simulink model "IndustrialMicrogrid"  (R2023a)
settings: Solver=FixedStepDiscrete  StartTime=0.0  StopTime=10  FixedStep=Ts  RelTol=1e-3
PostLoadFcn:
  | IndustrialMicrogridInputData
  | GfmGridFormingConverterInputParameters
model workspace (MAT data in the model file):
  caseNum = 2
undefined symbols (not defined in the file): base, BESS, DiscIntNeverNeededParam, grid, Grid, gridInverter, machine, microgrid, PV, PVInverter, PVTransformer, scrFactorRg, scrFactorXg, transformer, Ts
libraries: ee_lib x112, eeGeneralControl x104, nesl_utility_internal x64, simulink x56, nesl_utility x37, fl_lib x29, slpidlib x13, eeTransforms x11, eeTotalHarmonicDistorsion x8, eeRmsMeasurement x4, eeSinusoidalMeasurement x4, simulink_extras x2
(part 12 of 14)

== system IndustrialMicrogrid/MG2 Primary Substation/BESS and Controller 2/BESS/Grid-Forming Converter Control/Grid Voltage Reactive Power Support/Modifying Reactive Power Reference/Changing the Power Reference ==
  Vs : Inport
  Vd : Inport  Port=2
  Pref : Inport  Port=3
  Qref : Inport  Port=4
  Enable : EnablePort
  ActivePowerReference : Subsystem
  Constant1 : Constant  Value=voltreference*0.96
  EstimateIdForGivenIq : Subsystem
  EstimateIqForReactivePower : Subsystem
  Max : MinMax  Function=max  Inputs=2
  ReactivePowerReference : Subsystem
  Prefv : Outport
  Qrefv : Outport  Port=2
  wires:
  EstimateIqForReactivePower/1(Iq) -> EstimateIdForGivenIq/1(Iq), ReactivePowerReference/2(Iq)
  Constant1/1 -> EstimateIqForReactivePower/1(Vmin)
  Vs/1 -> ActivePowerReference/2(Vd), EstimateIqForReactivePower/3(Vs), ReactivePowerReference/1(Vd)
  EstimateIdForGivenIq/1(Id) -> ActivePowerReference/1(Id)
  Pref/1 -> ActivePowerReference/3(Pref)
  ActivePowerReference/1(PrefNew) -> Prefv/1
  ReactivePowerReference/1(QrefNew) -> Max/1
  Max/1 -> Qrefv/1
  Qref/1 -> Max/2
  Vd/1 -> EstimateIqForReactivePower/2(Vd)

== system IndustrialMicrogrid/MG2 Primary Substation/BESS and Controller 2/BESS/Grid-Forming Converter Control/Grid Voltage Reactive Power Support/Modifying Reactive Power Reference/Hysteresis ==
  Vs : Inport
  AND : Logic  IconShape=distinctive  AllPortsSameDT=off  OutDataTypeStr=boolean
  Compare To Constant : simulink/Logic and Bit Operations/Compare To Constant  relop=<  const=0.9  OutDataTypeStr=boolean
  Compare To Constant1 : simulink/Logic and Bit Operations/Compare To Constant  relop=<  const=0.95  OutDataTypeStr=boolean
  D Latch : simulink_extras/Flip Flops/D Latch
  OR : Logic  Operator=OR  IconShape=distinctive  AllPortsSameDT=off  OutDataTypeStr=boolean
  Terminator : Terminator
  LVFlag : Outport
  wires:
  Compare To Constant1/1 -> AND/1
  D Latch/1 -> AND/2
  AND/1 -> OR/1
  OR/1 -> LVFlag/1
  D Latch/2 -> Terminator/1
  Compare To Constant/1 -> D Latch/1, D Latch/2, OR/2
  Vs/1 -> Compare To Constant1/1, Compare To Constant/1

== system IndustrialMicrogrid/MG2 Primary Substation/BESS and Controller 2/BESS/Grid-Forming Converter Control/Grid Voltage Reactive Power Support/Modifying Reactive Power Reference/Not Altering the Power Reference ==
  Pref : Inport
  Qref : Inport  Port=2
  Enable : EnablePort
  Prefv : Outport
  Qrefv : Outport  Port=2
  wires:
  Pref/1 -> Prefv/1
  Qref/1 -> Qrefv/1

== system IndustrialMicrogrid/MG2 Primary Substation/BESS and Controller 2/BESS/Grid-Forming Converter Control/Measurement/Frequency Measurement/Frequency Measurement ==
  abc : Inport
  Constant : Constant
  Discrete-Time Integrator : DiscreteIntegrator  SampleTime=sampleTime  LimitOutput=on  ICPrevOutput=DiscIntNeverNeededParam  ICPrevScaledInput=DiscIntNeverNeededParam
  If : If  IfExpression=u1 > 0.9
  If Action Subsystem : Subsystem  TreatAsAtomicUnit=on
  If Action Subsystem1 : Subsystem  TreatAsAtomicUnit=on
  Merge : Merge
  Postive Sequence : Subsystem
  Freq : Outport
  wires:
  If/1 -> If Action Subsystem/Action
  If/2 -> If Action Subsystem1/Action
  Discrete-Time Integrator/1 -> If Action Subsystem/2(Time), If/1
  abc/1 -> Postive Sequence/1(abc)
  Constant/1 -> Discrete-Time Integrator/1
  If Action Subsystem/1(Freq) -> Merge/1
  If Action Subsystem1/1(Out1) -> Merge/2
  Merge/1 -> Freq/1
  Postive Sequence/1(posSeq) -> If Action Subsystem/1(V)

== system IndustrialMicrogrid/MG2 Primary Substation/BESS and Controller 2/BESS/Grid-Forming Converter Control/Measurement/abc2dq/Supply Current to dq ==
  abc : Inport
  Angle : Inport  Port=2
  Demux : Demux  Outputs=3
  Park Transform : eeTransforms/Park Transform  AxisAlignment=D-axis  PowerInvariant=off
  Terminator : Terminator
  Igd : Outport  VectorParamsAs1DForOutWhenUnconnected=off
  Igq : Outport  Port=2  VectorParamsAs1DForOutWhenUnconnected=off
  wires:
  Demux/3 -> Terminator/1
  Park Transform/1 -> Demux/1
  Demux/2 -> Igq/1
  Demux/1 -> Igd/1
  abc/1 -> Park Transform/1
  Angle/1 -> Park Transform/2

== system IndustrialMicrogrid/MG2 Primary Substation/BESS and Controller 2/BESS/Grid-Forming Converter Control/Measurement/abc2dq/Supply Voltage  to dq1 ==
  Angle : Inport
  abc : Inport  Port=2
  Demux : Demux  Outputs=3
  Park Transform : eeTransforms/Park Transform  AxisAlignment=D-axis  PowerInvariant=off
  Terminator : Terminator
  Vgd : Outport  VectorParamsAs1DForOutWhenUnconnected=off
  Vgq : Outport  Port=2  VectorParamsAs1DForOutWhenUnconnected=off
  wires:
  Demux/3 -> Terminator/1
  Park Transform/1 -> Demux/1
  Demux/2 -> Vgq/1
  Demux/1 -> Vgd/1
  abc/1 -> Park Transform/1
  Angle/1 -> Park Transform/2

== system IndustrialMicrogrid/MG2 Primary Substation/BESS and Controller 2/BESS/Grid-Forming Converter Control/Power Control/ActivePowerControl/droopControl ==
  Pref : Inport
  Pmeas : Inport  Port=2
  fref : Inport  Port=3
  cntrlflag : Inport  Port=4
  fgrid : Inport  Port=5
  Add : Sum  Inputs=+-
  Constant : Constant
  Constant5 : Constant  Value=pi/2
  Gain : Gain  Gain=powerFreq*2*pi
  Integrator with Wrapped State (Discrete or Continuous) : eeGeneralControl/Integrator with Wrapped State (Discrete or Continuous)  LabelModeActiveChoice=Discrete  WrappedStateUpperValue=2*pi  WrappedStateLowerValue=0  x0=0  Ts=activePowerSampleTime
      settings: LibrarySourceBlock=|
      | ee_sl_lib/General Control/Integrator with
      | Wrapped State
      | (Discrete or Continuous)
  Lead-Lag (Discrete or Continuous) : eeGeneralControl/Lead-Lag (Discrete or Continuous)  T1=droopT1  T2=droopT2  B=inf  A=-inf  init_option=Inherited from block input  x0=0  Ts=activePowerSampleTime
      settings: LibrarySourceBlock=|
      | ee_sl_lib/General Control/Lead-Lag
      | (Discrete or Continuous)
  Low-Pass Filter (Discrete or Continuous) : eeGeneralControl/Low-Pass Filter (Discrete or Continuous)  K=1  T=droopTC  B=inf  A=-inf  init_option=Specify as parameter  x0=0  Ts=activePowerSampleTime
  Sum : Sum  Inputs=|-+
  Sum1 : Sum  Inputs=|-+
  Terminator : Terminator
  Terminator1 : Terminator
  Terminator2 : Terminator
  mp : Gain  Gain=droopSlope
  Theta : Outport
  w : Outport  Port=2
  wires:
  Low-Pass Filter (Discrete or Continuous)/1 -> Sum1/1
  mp/1 -> Low-Pass Filter (Discrete or Continuous)/1
  Sum/1 -> mp/1
  Pmeas/1 -> Lead-Lag (Discrete or Continuous)/1
  Add/1 -> Theta/1
  Constant5/1 -> Add/2
  Pref/1 -> Sum/1
  Gain/1 -> Integrator with Wrapped State (Discrete or Continuous)/1, w/1
  Lead-Lag (Discrete or Continuous)/1 -> Sum/2
  Integrator with Wrapped State (Discrete or Continuous)/1 -> Add/1
  Constant/1 -> Sum1/2
  Sum1/1 -> Gain/1
  fgrid/1 -> Terminator/1
  fref/1 -> Terminator1/1
  cntrlflag/1 -> Terminator2/1

== system IndustrialMicrogrid/MG2 Primary Substation/BESS and Controller 2/BESS/Grid-Forming Converter Control/Power Control/ActivePowerControl/vsmControl ==
  note: Measured power
  note: Damping power input
  Pref : Inport
  Pmeas : Inport  Port=2
  fref : Inport  Port=3
  cntrlflag : Inport  Port=4
  fgrid : Inport  Port=5
  Add : Sum  Inputs=+-
  Constant2 : Constant  Value=pi/2
  Damping Frequency : Subsystem  Variant=on  VariantControlMode=label  VariantControl=Choice  LabelModeActiveChoice=constFreq
  Discrete-Time Integrator : DiscreteIntegrator  IntegratorMethod=Integration: Backward Euler  InitialCondition=1  SampleTime=activePowerSampleTime  LimitOutput=on  UpperSaturationLimit=1.1  LowerSaturationLimit=0.9  ICPrevOutput=DiscIntNeverNeededParam  ICPrevScaledInput=DiscIntNeverNeededParam
  Gain : Gain  Gain=powerFreq*2*pi
  Gain1 : Gain  Gain=1/vsmInertiaTC
  Gain2 : Gain  Gain=vsmDampingConst*powerFreq
  Integrator with Wrapped State (Discrete or Continuous) : eeGeneralControl/Integrator with Wrapped State (Discrete or Continuous)  LabelModeActiveChoice=Discrete  WrappedStateUpperValue=2*pi  WrappedStateLowerValue=0  x0=0  Ts=activePowerSampleTime
      settings: LibrarySourceBlock=|
      | ee_sl_lib/General Control/Integrator with
      | Wrapped State
      | (Discrete or Continuous)
  Low-Pass Filter (Discrete or Continuous) : eeGeneralControl/Low-Pass Filter (Discrete or Continuous)  K=1  T=vsmPmeasFilterTC  B=inf  A=-inf  init_option=Specify as parameter  x0=0  Ts=activePowerSampleTime
  Power Reference Selection : Subsystem
  Saturation : Saturate  UpperLimit=dampingPowerMaxLimit  LowerLimit=dampingPowerMinLimit
  Sum1 : Sum  Inputs=-+-|
  Sum2 : Sum  Inputs=|+-
  Unit Delay : UnitDelay  SampleTime=-1  HasFrameUpgradeWarning=on
  Unit Delay1 : UnitDelay  SampleTime=-1  HasFrameUpgradeWarning=on
  Theta : Outport
  w : Outport  Port=2
  wires:
  Integrator with Wrapped State (Discrete or Continuous)/1 -> Add/1
  Sum1/1 -> Gain1/1  "Pinertia"
  Constant2/1 -> Add/2
  Add/1 -> Theta/1
  Discrete-Time Integrator/1 -> Gain/1, Unit Delay1/1, Sum2/1
  Low-Pass Filter (Discrete or Continuous)/1 -> Sum1/1
  Gain2/1 -> Saturation/1
  Power Reference Selection/1(power) -> Sum1/2
  Sum2/1 -> Unit Delay/1
  Gain1/1 -> Discrete-Time Integrator/1
  Gain/1 -> Integrator with Wrapped State (Discrete or Continuous)/1, w/1
  Unit Delay/1 -> Gain2/1
  Unit Delay1/1 -> [Wsm]
  Saturation/1 -> Sum1/3  "Pdamping"
  fgrid/1 -> Damping Frequency/1(fref)
  Damping Frequency/1(fmeas) -> Sum2/2
  cntrlflag/1 -> Power Reference Selection/1(cntrlflag)
  Pref/1 -> Power Reference Selection/2(Pref)
  fref/1 -> Power Reference Selection/3(fref)
  Pmeas/1 -> Low-Pass Filter (Discrete or Continuous)/1
  [Wsm] -> Power Reference Selection/4(Wsm)

== system IndustrialMicrogrid/MG2 Primary Substation/BESS and Controller 2/BESS/Grid-Forming Converter Control/Power Control/ReactiveControl/Voltage  Reference Selection ==
  cntrlflag : Inport
  Qref : Inport  Port=2
  Qmeas : Inport  Port=3
  Vref : Inport  Port=4
  Vgdmeas : Inport  Port=5
  If : If
  If Action Subsystem : Subsystem  TreatAsAtomicUnit=on
  If Action Subsystem1 : Subsystem  TreatAsAtomicUnit=on
  Merge : Merge
  Rate Transition : RateTransition
  Vd : Outport
  wires:
  If/1 -> If Action Subsystem/Action
  If Action Subsystem/1(Vd) -> Merge/1
  If/2 -> If Action Subsystem1/Action
  cntrlflag/1 -> Rate Transition/1
  Merge/1 -> Vd/1
  Qmeas/1 -> If Action Subsystem/2(Qmeas)
  Qref/1 -> If Action Subsystem/1(Qref)
  If Action Subsystem1/1(Voltage) -> Merge/2
  Vref/1 -> If Action Subsystem1/1(Vref)
  Vgdmeas/1 -> If Action Subsystem1/2(Vmeas)
  Rate Transition/1 -> If/1

== system IndustrialMicrogrid/MG2 Primary Substation/BESS and Controller 2/BESS/Grid-Forming Converter Control/VoltageCurrentControl/Controller/Id Current Limiting ==
  Imax : Inport
  Id : Inport  Port=2
  Abs : Abs  SaturateOnIntegerOverflow=off
  Switch : Switch  Criteria=u2 > Threshold  SaturateOnIntegerOverflow=off  InputSameDT=off
  Idref : Outport
  wires:
  Id/1 -> Switch/3
  Abs/1 -> Switch/2
  Imax/1 -> Abs/1, Switch/1
  Switch/1 -> Idref/1

== system IndustrialMicrogrid/MG2 Primary Substation/BESS and Controller 2/BESS/Grid-Forming Converter Control/VoltageCurrentControl/Controller/Iq Current Limiting ==
  Imax : Inport
  Iq : Inport  Port=2
  Abs : Abs  SaturateOnIntegerOverflow=off
  Switch : Switch  Criteria=u2 > Threshold  SaturateOnIntegerOverflow=off  InputSameDT=off
  Iqref : Outport
  wires:
  Iq/1 -> Switch/3
  Abs/1 -> Switch/2
  Imax/1 -> Abs/1, Switch/1
  Switch/1 -> Iqref/1

== system IndustrialMicrogrid/MG2 Primary Substation/BESS and Controller 2/BESS/Grid-Forming Converter Control/VoltageCurrentControl/Controller/Voltage control ==
  e : Inport
  resetBlackStart : Inport  Port=2
  Discrete-Time Integrator : DiscreteIntegrator  IntegratorMethod=Integration: Backward Euler  ExternalReset=level  SampleTime=voltControlTs  LimitOutput=on  UpperSaturationLimit=VdMaxCt  LowerSaturationLimit=VdMinCt  ICPrevOutput=DiscIntNeverNeededParam  ICPrevScaledInput=DiscIntNeverNeededParam
  Ki : Gain  Gain=VdIGain
  Kp : Gain  Gain=vdPGain
  Limit : Saturate  UpperLimit=VdMaxCt  LowerLimit=VdMinCt
  Sum7 : Sum  Inputs=|++
  u : Outport  VectorParamsAs1DForOutWhenUnconnected=off
  wires:
  Discrete-Time Integrator/1 -> Sum7/2
  Kp/1 -> Sum7/1
  Limit/1 -> u/1
  Ki/1 -> Discrete-Time Integrator/1
  Sum7/1 -> Limit/1
  e/1 -> Kp/1, Ki/1
  resetBlackStart/1 -> Discrete-Time Integrator/2

== system IndustrialMicrogrid/MG2 Primary Substation/BESS and Controller 2/BESS/Grid-Forming Converter Control/VoltageCurrentControl/Controller/Voltage control1 ==
  e : Inport
  resetBlackStart : Inport  Port=2
  Discrete-Time Integrator : DiscreteIntegrator  IntegratorMethod=Integration: Backward Euler  ExternalReset=level  SampleTime=voltControlTs  LimitOutput=on  UpperSaturationLimit=VqMaxCt  LowerSaturationLimit=VqMinCt  ICPrevOutput=DiscIntNeverNeededParam  ICPrevScaledInput=DiscIntNeverNeededParam
  Ki : Gain  Gain=VqIGain
  Kp : Gain  Gain=VqPGain
  Limit : Saturate  UpperLimit=VqMaxCt  LowerLimit=VqMinCt
  Sum7 : Sum  Inputs=|++
  u : Outport  VectorParamsAs1DForOutWhenUnconnected=off
  wires:
  Discrete-Time Integrator/1 -> Sum7/2
  Sum7/1 -> Limit/1
  e/1 -> Ki/1, Kp/1
  Kp/1 -> Sum7/1
  Ki/1 -> Discrete-Time Integrator/1
  Limit/1 -> u/1
  resetBlackStart/1 -> Discrete-Time Integrator/2

== system IndustrialMicrogrid/MG2 Primary Substation/BESS and Controller 2/BESS/Grid-Forming Converter Control/VoltageCurrentControl/Controller/d-axis current control ==
  e : Inport
  resetBlackStart : Inport  Port=2
  Discrete-Time Integrator : DiscreteIntegrator  IntegratorMethod=Integration: Backward Euler  ExternalReset=level  SampleTime=currentControlTs  LimitOutput=on  UpperSaturationLimit=4  LowerSaturationLimit=-4  ICPrevOutput=DiscIntNeverNeededParam  ICPrevScaledInput=DiscIntNeverNeededParam
  Ki : Gain  Gain=IdIGain
  Kp : Gain  Gain=IdPGain
  Limit : Saturate  UpperLimit=4  LowerLimit=-4
  Sum7 : Sum  Inputs=|++
  u : Outport  VectorParamsAs1DForOutWhenUnconnected=off
  wires:
  Discrete-Time Integrator/1 -> Sum7/2
  Sum7/1 -> Limit/1
  e/1 -> Ki/1, Kp/1
  Kp/1 -> Sum7/1
  Limit/1 -> u/1
  Ki/1 -> Discrete-Time Integrator/1
  resetBlackStart/1 -> Discrete-Time Integrator/2

== system IndustrialMicrogrid/MG2 Primary Substation/BESS and Controller 2/BESS/Grid-Forming Converter Control/VoltageCurrentControl/Controller/q-axis current control ==
  e : Inport
  resetBlackStart : Inport  Port=2
  Discrete-Time Integrator : DiscreteIntegrator  IntegratorMethod=Integration: Backward Euler  ExternalReset=level  SampleTime=currentControlTs  LimitOutput=on  UpperSaturationLimit=3  LowerSaturationLimit=-3  ICPrevOutput=DiscIntNeverNeededParam  ICPrevScaledInput=DiscIntNeverNeededParam
  Ki : Gain  Gain=IqIGain
  Kp : Gain  Gain=IqPGain
  Limit : Saturate  UpperLimit=3  LowerLimit=-3
  Sum7 : Sum  Inputs=|++
  u : Outport  VectorParamsAs1DForOutWhenUnconnected=off
  wires:
  Ki/1 -> Discrete-Time Integrator/1
  Kp/1 -> Sum7/1
  e/1 -> Kp/1, Ki/1
  Sum7/1 -> Limit/1
  Limit/1 -> u/1
  Discrete-Time Integrator/1 -> Sum7/2
  resetBlackStart/1 -> Discrete-Time Integrator/2

== system IndustrialMicrogrid/Operator Room/OperatorControlRoom/MG1 Controller : Commands and Measurements/Microgrid Controller 1 : Commands and Measurements/Measurements and visualizations /BESS, PV and Load Measurements/Active and reactive Power ==
  Grid Active Power : Inport
  BESS Active Power : Inport  Port=2
  Load Active Power : Inport  Port=3
  Grid Reactive Power : Inport  Port=4
  BESS Reactive Power : Inport  Port=5
  Load Reactive Power : Inport  Port=6
  Bus Creator : BusCreator  Inputs=3
  Bus Creator1 : BusCreator  Inputs=3
  Power  Measurements : Scope  NumInputPorts=2
  Active Power : Outport
  Reactive Power : Outport  Port=2
  wires:
  BESS Active Power/1 -> Bus Creator/2
  BESS Reactive Power/1 -> Bus Creator1/2
  Bus Creator1/1 -> Reactive Power/1, Power  Measurements/2
  Bus Creator/1 -> Active Power/1, Power  Measurements/1
  Grid Active Power/1 -> Bus Creator/1
  Load Active Power/1 -> Bus Creator/3
  Grid Reactive Power/1 -> Bus Creator1/1
  Load Reactive Power/1 -> Bus Creator1/3

== system IndustrialMicrogrid/Operator Room/OperatorControlRoom/MG1 Controller : Commands and Measurements/Microgrid Controller 1 : Commands and Measurements/Measurements and visualizations /BESS, PV and Load Measurements/BESS and PV Measurements ==
  Vabc : Inport
  Iabc : Inport  Port=2
  BESS Measurements : Scope  NumInputPorts=4
  Iabc1 : InportShadow  Port=2
  "Inverter Active & Reactive Power " : Subsystem
  Vabc1 : InportShadow
  wires:
  "Inverter Active & Reactive Power "/2(Q) -> BESS Measurements/2  "BESS  Reactive Power (pu)"
  Vabc1/1 -> BESS Measurements/3  "BESS Voltage (pu)"
  "Inverter Active & Reactive Power "/1(P) -> BESS Measurements/1  "BESS  Active Power (pu)"
  Iabc/1 -> "Inverter Active & Reactive Power "/2(Iabc)  "BESS Current (pu)"
  Vabc/1 -> "Inverter Active & Reactive Power "/1(Vabc)  "BESS Voltage (pu)"
  Iabc1/1 -> BESS Measurements/4  "BESS Current (pu)"

== system IndustrialMicrogrid/Operator Room/OperatorControlRoom/MG1 Controller : Commands and Measurements/Microgrid Controller 1 : Commands and Measurements/Measurements and visualizations /BESS, PV and Load Measurements/Load Measurements ==
  Load Active Power : Inport
  Load Reactive Power : Inport  Port=2
  Load Current(p.u.) : Inport  Port=3
  Load Voltage (p.u.) : Inport  Port=4
  Load Voltage RMS (p.u.) : Inport  Port=5
  Bus Creator4 : BusCreator  Inputs=2
  Load Measurements : Scope  NumInputPorts=4
  wires:
  Load Current(p.u.)/1 -> Load Measurements/2  "Load Current(p.u.)"
  Bus Creator4/1 -> Load Measurements/1  "Load Active Power (kW) and reactive power (KVAr)"
  Load Reactive Power/1 -> Bus Creator4/2  "Load Reactive Power (KVAr)"
  Load Voltage RMS (p.u.)/1 -> Load Measurements/4  "Load Voltage RMS (p.u.)"
  Load Active Power/1 -> Bus Creator4/1  "Load Active Power (KW)"
  Load Voltage (p.u.)/1 -> Load Measurements/3  "Load Voltage (p.u.)"

== system IndustrialMicrogrid/Operator Room/OperatorControlRoom/MG1 Controller : Commands and Measurements/Microgrid Controller 1 : Commands and Measurements/Measurements and visualizations /Resynchronization and Planned Islanding/Planned Islanding ==
  Grid Frequency : Inport
  Island Frequency : Inport  Port=2
  Grid Current : Inport  Port=3
  Island Voltage : Inport  Port=4
  Grid Voltage1 : Inport  Port=5
  PlannedIslandCommand : Inport  Port=6
  PlannedIsland : Inport  Port=7
  Power Tracking Command : Inport  Port=8
  " Grid and Island Voltage Frequency " : Scope  NumInputPorts=2
  Bus Creator1 : BusCreator  Inputs=2
  Bus Creator2 : BusCreator  Inputs=2
  Bus Creator3 : BusCreator  Inputs=3
  Bus Creator4 : BusCreator  Inputs=2
  "Grid Active & Reactive Power " : Subsystem
  Grid Voltage2 : InportShadow  Port=5
  Planned Islanding PCC voltage,Current : Scope  NumInputPorts=4
  wires:
  Bus Creator4/1 -> Planned Islanding PCC voltage,Current/4
  Bus Creator3/1 -> Planned Islanding PCC voltage,Current/1
  PlannedIslandCommand/1 -> Bus Creator3/1
  Grid Voltage2/1 -> Planned Islanding PCC voltage,Current/3, "Grid Active & Reactive Power "/1(Vabc)  "Grid Voltage"
  "Grid Active & Reactive Power "/2(Q) -> Bus Creator4/2  "Reactive Power (pu)"
  Grid Current/1 -> Planned Islanding PCC voltage,Current/2, "Grid Active & Reactive Power "/2(Iabc)
  "Grid Active & Reactive Power "/1(P) -> Bus Creator4/1  "Active Power (pu)"
  PlannedIsland/1 -> Bus Creator3/2
  Grid Frequency/1 -> Bus Creator1/1  "Grid Frequency"
  Island Frequency/1 -> Bus Creator1/2  "Island Frequency"
  Bus Creator1/1 -> " Grid and Island Voltage Frequency "/1
  Bus Creator2/1 -> " Grid and Island Voltage Frequency "/2
  Grid Voltage1/1 -> Bus Creator2/1  "Grid Voltage"
  Island Voltage/1 -> Bus Creator2/2  "Island Voltage"
  Power Tracking Command/1 -> Bus Creator3/3

== system IndustrialMicrogrid/Operator Room/OperatorControlRoom/MG1 Controller : Commands and Measurements/Microgrid Controller 1 : Commands and Measurements/Measurements and visualizations /Resynchronization and Planned Islanding/Resync ==
  Grid Frequency : Inport
  Island Frequency : Inport  Port=2
  ResynchCommand : Inport  Port=3
  Grid Angle : Inport  Port=4
  Island Angle : Inport  Port=5
  Resynchronization : Inport  Port=6
  Grid Voltage : Inport  Port=7
  Grid Current : Inport  Port=8
  Island Voltage : Inport  Port=9
  Frequency Error : Inport  Port=10
  Grid Voltage1 : Inport  Port=11
  Phase Angle Error : Inport  Port=12
  Voltage Error : Inport  Port=13
  Bus Creator{,1..4} (5 alike) : BusCreator  Inputs=2
  "Grid Active & Reactive Power " : Subsystem
  Resynch and PCC voltage,Current : Scope  NumInputPorts=4
  Voltage and Frequency Matching : Scope  NumInputPorts=6
  wires:
  Grid Current/1 -> "Grid Active & Reactive Power "/2(Iabc), Resynch and PCC voltage,Current/2
  Bus Creator1/1 -> Voltage and Frequency Matching/2
  Resynchronization/1 -> Bus Creator3/2
  Bus Creator3/1 -> Resynch and PCC voltage,Current/1
  "Grid Active & Reactive Power "/1(P) -> Bus Creator4/1  "Active Power (pu)"
  Island Voltage/1 -> Bus Creator2/2
  Grid Voltage1/1 -> Resynch and PCC voltage,Current/3, "Grid Active & Reactive Power "/1(Vabc)
  Bus Creator4/1 -> Resynch and PCC voltage,Current/4
  Bus Creator2/1 -> Voltage and Frequency Matching/3
  Bus Creator/1 -> Voltage and Frequency Matching/1
  Grid Frequency/1 -> Bus Creator/1
  Grid Angle/1 -> Bus Creator1/1
  Voltage Error/1 -> Voltage and Frequency Matching/6
  Island Frequency/1 -> Bus Creator/2
  Island Angle/1 -> Bus Creator1/2
  Phase Angle Error/1 -> Voltage and Frequency Matching/5
  Grid Voltage/1 -> Bus Creator2/1
  "Grid Active & Reactive Power "/2(Q) -> Bus Creator4/2  "Reactive Power (pu)"
  ResynchCommand/1 -> Bus Creator3/1
  Frequency Error/1 -> Voltage and Frequency Matching/4

== system IndustrialMicrogrid/Operator Room/OperatorControlRoom/MG1 Controller : Commands and Measurements/Microgrid Controller 1 : Commands and Measurements/Monitoring of system performance/Load /Subsystem4 ==
  u : Inport
  Change Detector : eeGeneralControl/Change Detector  VariantControl=Variant1  LabelModeActiveChoice=Discrete  ChangeType=Rising edge  x0=0  Ts=Ts
      settings: LibrarySourceBlock=ee_sl_lib/General Control/Change Detector
  Change Detector1 : eeGeneralControl/Change Detector  VariantControl=Variant1  LabelModeActiveChoice=Discrete  ChangeType=Rising edge  x0=0  Ts=Ts
      settings: LibrarySourceBlock=ee_sl_lib/General Control/Change Detector
  Compare To Constant2 : simulink/Logic and Bit Operations/Compare To Constant  relop=<=  const=microgrid.loadVolatgeRMSLow  OutDataTypeStr=boolean
  Compare To Constant3 : simulink/Logic and Bit Operations/Compare To Constant  relop=>  const=microgrid.loadVolatgeRMSHigh  OutDataTypeStr=boolean
  Out1 : Outport
  Out2 : Outport  Port=2
  wires:
  Change Detector/1 -> Out1/1
  Compare To Constant2/1 -> Change Detector/1
  u/1 -> Compare To Constant3/1, Compare To Constant2/1
  Change Detector1/1 -> Out2/1
  Compare To Constant3/1 -> Change Detector1/1

== system IndustrialMicrogrid/Operator Room/OperatorControlRoom/MG1 Controller : Commands and Measurements/Microgrid Controller 1 : Commands and Measurements/Monitoring of system performance/Load /start at 0.2 s2 ==
  In1 : Inport
  Constant : Constant  Value=0.707
  Step : Step  Time=0.3  SampleTime=Ts
  Switch : Switch  Criteria=u2 > Threshold  Threshold=0.5  SaturateOnIntegerOverflow=off  InputSameDT=off
  u : Outport
  wires:
  In1/1 -> Switch/1
  Switch/1 -> u/1
  Constant/1 -> Switch/3
  Step/1 -> Switch/2

== system IndustrialMicrogrid/Operator Room/OperatorControlRoom/MG1 Controller : Commands and Measurements/Microgrid Controller 1 : Commands and Measurements/Monitoring of system performance/Load /start at 0.2 s4 ==
  In1 : Inport
  Constant : Constant  Value=0.491
  Step : Step  Time=0.3  SampleTime=Ts
  Switch : Switch  Criteria=u2 > Threshold  Threshold=0.5  SaturateOnIntegerOverflow=off  InputSameDT=off
  u : Outport
  wires:
  In1/1 -> Switch/1
  Switch/1 -> u/1
  Constant/1 -> Switch/3
  Step/1 -> Switch/2

== system IndustrialMicrogrid/Operator Room/OperatorControlRoom/MG1 Controller : Commands and Measurements/Microgrid Controller 1 : Commands and Measurements/Monitoring of system performance/Load /start at 0.2 s5 ==
  In1 : Inport
  Constant : Constant  Value=75
  Step : Step  Time=0.3  SampleTime=Ts
  Switch : Switch  Criteria=u2 > Threshold  Threshold=0.5  SaturateOnIntegerOverflow=off  InputSameDT=off
  u : Outport
  wires:
  Step/1 -> Switch/2
  Constant/1 -> Switch/3
  Switch/1 -> u/1
  In1/1 -> Switch/1

== system IndustrialMicrogrid/Operator Room/OperatorControlRoom/MG1 Controller : Commands and Measurements/Microgrid Controller 1 : Commands and Measurements/Monitoring of system performance/Microgrid/Subsystem ==
  u : Inport
  Change Detector : eeGeneralControl/Change Detector  VariantControl=Variant1  LabelModeActiveChoice=Discrete  ChangeType=Rising edge  x0=0  Ts=Ts
      settings: LibrarySourceBlock=ee_sl_lib/General Control/Change Detector
  Change Detector1 : eeGeneralControl/Change Detector  VariantControl=Variant1  LabelModeActiveChoice=Discrete  ChangeType=Rising edge  x0=0  Ts=Ts
      settings: LibrarySourceBlock=ee_sl_lib/General Control/Change Detector
  Compare To Constant2 : simulink/Logic and Bit Operations/Compare To Constant  relop=<  const=microgrid.frequencyLow  OutDataTypeStr=boolean
  Compare To Constant3 : simulink/Logic and Bit Operations/Compare To Constant  relop=>  const=microgrid.frequencyHigh  OutDataTypeStr=boolean
  Out1 : Outport
  Out2 : Outport  Port=2
  wires:
  Change Detector/1 -> Out1/1
  Compare To Constant2/1 -> Change Detector/1
  u/1 -> Compare To Constant3/1, Compare To Constant2/1
  Change Detector1/1 -> Out2/1
  Compare To Constant3/1 -> Change Detector1/1

== system IndustrialMicrogrid/Operator Room/OperatorControlRoom/MG1 Controller : Commands and Measurements/Microgrid Controller 1 : Commands and Measurements/Monitoring of system performance/Microgrid/Subsystem3 ==
  u : Inport
  Change Detector : eeGeneralControl/Change Detector  VariantControl=Variant1  LabelModeActiveChoice=Discrete  ChangeType=Rising edge  x0=0  Ts=Ts
      settings: LibrarySourceBlock=ee_sl_lib/General Control/Change Detector
  Change Detector1 : eeGeneralControl/Change Detector  VariantControl=Variant1  LabelModeActiveChoice=Discrete  ChangeType=Rising edge  x0=0  Ts=Ts
      settings: LibrarySourceBlock=ee_sl_lib/General Control/Change Detector
  Compare To Constant2 : simulink/Logic and Bit Operations/Compare To Constant  relop=<=  const=microgrid.voltageLow  OutDataTypeStr=boolean
  Compare To Constant3 : simulink/Logic and Bit Operations/Compare To Constant  relop=>  const=microgrid.voltageHigh  OutDataTypeStr=boolean
  Out1 : Outport
  Out2 : Outport  Port=2
  wires:
  Compare To Constant3/1 -> Change Detector1/1
  Change Detector1/1 -> Out2/1
  u/1 -> Compare To Constant2/1, Compare To Constant3/1
  Compare To Constant2/1 -> Change Detector/1
  Change Detector/1 -> Out1/1

== system IndustrialMicrogrid/Operator Room/OperatorControlRoom/MG1 Controller : Commands and Measurements/Microgrid Controller 1 : Commands and Measurements/Monitoring of system performance/Microgrid/start at 0.2 s1 ==
  In1 : Inport
  Constant : Constant
  Step : Step  Time=0.3  SampleTime=Ts
  Switch : Switch  Criteria=u2 > Threshold  Threshold=0.5  SaturateOnIntegerOverflow=off  InputSameDT=off
  u : Outport
  wires:
  Step/1 -> Switch/2
  Constant/1 -> Switch/3
  Switch/1 -> u/1
  In1/1 -> Switch/1

== system IndustrialMicrogrid/Operator Room/OperatorControlRoom/MG1 Controller : Commands and Measurements/Microgrid Controller 1 : Commands and Measurements/Monitoring of system performance/Microgrid/start at 0.2 s3 ==
  In1 : Inport
  Constant : Constant  Value=60
  Step : Step  Time=0.3  SampleTime=Ts
  Switch : Switch  Criteria=u2 > Threshold  Threshold=0.5  SaturateOnIntegerOverflow=off  InputSameDT=off
  u : Outport
  wires:
  Step/1 -> Switch/2
  Constant/1 -> Switch/3
  Switch/1 -> u/1
  In1/1 -> Switch/1

== system IndustrialMicrogrid/Operator Room/OperatorControlRoom/MG1 Controller : Commands and Measurements/Microgrid Controller 1 : Commands and Measurements/Monitoring of system performance/Subsystem/start at 2.5 s ==
  ReactivePower : Inport
  Constant : Constant  Value=0
  Step : Step  Time=2.5  SampleTime=Ts
  Switch : Switch  Criteria=u2 > Threshold  Threshold=0.5  SaturateOnIntegerOverflow=off  InputSameDT=off
  u : Outport
  wires:
  ReactivePower/1 -> Switch/1
  Switch/1 -> u/1
  Constant/1 -> Switch/3
  Step/1 -> Switch/2

== system IndustrialMicrogrid/Operator Room/OperatorControlRoom/MG1 Controller : Commands and Measurements/Microgrid Controller 1 : Commands and Measurements/Monitoring of system performance/Subsystem/start at 2.5 s1 ==
  ActivePower : Inport
  Constant : Constant  Value=0
  Step : Step  Time=2.5  SampleTime=Ts
  Switch : Switch  Criteria=u2 > Threshold  Threshold=0.5  SaturateOnIntegerOverflow=off  InputSameDT=off
  u : Outport
  wires:
  Step/1 -> Switch/2
  Constant/1 -> Switch/3
  Switch/1 -> u/1
  ActivePower/1 -> Switch/1

== system IndustrialMicrogrid/Operator Room/OperatorControlRoom/MG2 Controller : Commands and Measurements/Microgrid Controller 2 : Commands and Measurements/Measurements and visualizations 1/BESS, PV and Load Measurements/Active and reactive Power ==
  Grid Active Power : Inport
  BESS Active Power : Inport  Port=2
  Load Active Power : Inport  Port=3
  PV Active Power : Inport  Port=4
  Grid Reactive Power : Inport  Port=5
  BESS Reactive Power : Inport  Port=6
  Load Reactive Power : Inport  Port=7
  PV Reactive Power : Inport  Port=8
  Diesel Reactive Power : Inport  Port=9
  Diesel Active Power : Inport  Port=10
  Bus Creator : BusCreator  Inputs=5
  Bus Creator1 : BusCreator  Inputs=5
  Power  Measurements : Scope  NumInputPorts=2
  Active Power : Outport
  Reactive Power : Outport  Port=2
  wires:
  BESS Active Power/1 -> Bus Creator/2
  BESS Reactive Power/1 -> Bus Creator1/2
  Bus Creator1/1 -> Reactive Power/1, Power  Measurements/2
  Bus Creator/1 -> Active Power/1, Power  Measurements/1
  Grid Active Power/1 -> Bus Creator/1
  PV Active Power/1 -> Bus Creator/4
  Load Active Power/1 -> Bus Creator/3
  Grid Reactive Power/1 -> Bus Creator1/1
  Load Reactive Power/1 -> Bus Creator1/3
  PV Reactive Power/1 -> Bus Creator1/4
  Diesel Reactive Power/1 -> Bus Creator1/5
  Diesel Active Power/1 -> Bus Creator/5

== system IndustrialMicrogrid/Operator Room/OperatorControlRoom/MG2 Controller : Commands and Measurements/Microgrid Controller 2 : Commands and Measurements/Measurements and visualizations 1/BESS, PV and Load Measurements/BESS and PV Measurements ==
  Vpv (V) : Inport
  Vabc : Inport  Port=2
  Iabc : Inport  Port=3
  Ipv (A) : Inport  Port=4
  PV Active Power : Inport  Port=5
  PV Reactive Power : Inport  Port=6
  BESS Measurements : Scope  NumInputPorts=4
  Iabc1 : InportShadow  Port=3
  "Inverter Active & Reactive Power " : Subsystem
  PV Measurmeents : Scope  NumInputPorts=4
  Vabc1 : InportShadow  Port=2
  wires:
  Vpv (V)/1 -> PV Measurmeents/1  "PV Voltage (pu)"
  "Inverter Active & Reactive Power "/2(Q) -> BESS Measurements/2  "BESS  Reactive Power (pu)"
  Vabc1/1 -> BESS Measurements/3  "BESS Voltage (pu)"
  Ipv (A)/1 -> PV Measurmeents/2  "PV Current (pu)"
  "Inverter Active & Reactive Power "/1(P) -> BESS Measurements/1  "BESS  Active Power (pu)"
  Iabc/1 -> "Inverter Active & Reactive Power "/2(Iabc)  "BESS Current (pu)"
  Vabc/1 -> "Inverter Active & Reactive Power "/1(Vabc)  "BESS Voltage (pu)"
  Iabc1/1 -> BESS Measurements/4  "BESS Current (pu)"
  PV Active Power/1 -> PV Measurmeents/3  "PV Active Power (MW)"
  PV Reactive Power/1 -> PV Measurmeents/4  "PV Rective Power (MVAr)"

== system IndustrialMicrogrid/Operator Room/OperatorControlRoom/MG2 Controller : Commands and Measurements/Microgrid Controller 2 : Commands and Measurements/Measurements and visualizations 1/BESS, PV and Load Measurements/Load Measurements ==
  Load Active Power : Inport
  Load Reactive Power : Inport  Port=2
  Load Current(p.u.) : Inport  Port=3
  Load Voltage (p.u.) : Inport  Port=4
  Load Voltage RMS (p.u.) : Inport  Port=5
  Bus Creator4 : BusCreator  Inputs=2
  Load Measurements : Scope  NumInputPorts=4
  wires:
  Load Current(p.u.)/1 -> Load Measurements/2  "Load Current(p.u.)"
  Bus Creator4/1 -> Load Measurements/1  "Load Active Power (kW) and reactive power (KVAr)"
  Load Reactive Power/1 -> Bus Creator4/2  "Load Reactive Power (KVAr)"
  Load Voltage RMS (p.u.)/1 -> Load Measurements/4  "Load Voltage RMS (p.u.)"
  Load Active Power/1 -> Bus Creator4/1  "Load Active Power (KW)"
  Load Voltage (p.u.)/1 -> Load Measurements/3  "Load Voltage (p.u.)"

== system IndustrialMicrogrid/Operator Room/OperatorControlRoom/MG2 Controller : Commands and Measurements/Microgrid Controller 2 : Commands and Measurements/Measurements and visualizations 1/Resynchronization and Planned Islanding/Planned Islanding ==
  Grid Frequency : Inport
  Island Frequency : Inport  Port=2
  Grid Current : Inport  Port=3
  Island Voltage : Inport  Port=4
  Grid Voltage1 : Inport  Port=5
  PlannedIslandCommand : Inport  Port=6
  PlannedIsland : Inport  Port=7
  Power Tracking Command : Inport  Port=8
  Grid Voltage abc : Inport  Port=9
  " Grid and Island Voltage Frequency " : Scope  NumInputPorts=2
  Bus Creator1 : BusCreator  Inputs=2
  Bus Creator2 : BusCreator  Inputs=2
  Bus Creator3 : BusCreator  Inputs=3
  Bus Creator4 : BusCreator  Inputs=2
  "Grid Active & Reactive Power " : Subsystem
  Planned Islanding PCC voltage,Current : Scope  NumInputPorts=4
  wires:
  Power Tracking Command/1 -> Bus Creator3/3
  Island Voltage/1 -> Bus Creator2/2  "Island Voltage"
  Grid Voltage1/1 -> Bus Creator2/1  "Grid Voltage"
  Bus Creator2/1 -> " Grid and Island Voltage Frequency "/2
  Bus Creator1/1 -> " Grid and Island Voltage Frequency "/1
  Island Frequency/1 -> Bus Creator1/2  "Island Frequency"
  Grid Frequency/1 -> Bus Creator1/1  "Grid Frequency"
  PlannedIsland/1 -> Bus Creator3/2
  "Grid Active & Reactive Power "/1(P) -> Bus Creator4/1  "Active Power (pu)"
  Grid Current/1 -> "Grid Active & Reactive Power "/2(Iabc), Planned Islanding PCC voltage,Current/2
  "Grid Active & Reactive Power "/2(Q) -> Bus Creator4/2  "Reactive Power (pu)"
  Grid Voltage abc/1 -> "Grid Active & Reactive Power "/1(Vabc), Planned Islanding PCC voltage,Current/3  "Grid Voltage"
  PlannedIslandCommand/1 -> Bus Creator3/1
  Bus Creator3/1 -> Planned Islanding PCC voltage,Current/1
  Bus Creator4/1 -> Planned Islanding PCC voltage,Current/4

== system IndustrialMicrogrid/Operator Room/OperatorControlRoom/MG2 Controller : Commands and Measurements/Microgrid Controller 2 : Commands and Measurements/Measurements and visualizations 1/Resynchronization and Planned Islanding/Resync ==
  Grid Frequency : Inport
  Island Frequency : Inport  Port=2
  In1 : Inport  Port=3
  Grid Angle : Inport  Port=4
  Island Angle : Inport  Port=5
  Resynchronization : Inport  Port=6
  Grid Voltage : Inport  Port=7
  Grid Current : Inport  Port=8
  Island Voltage : Inport  Port=9
  Frequency Error : Inport  Port=10
  Grid Voltage abc : Inport  Port=11
  Phase Angle Error : Inport  Port=12
  Voltage Error : Inport  Port=13
  Bus Creator{,1..4} (5 alike) : BusCreator  Inputs=2
  "Grid Active & Reactive Power " : Subsystem
  Resynch and PCC voltage,Current : Scope  NumInputPorts=4
  Voltage and Frequency Matching : Scope  NumInputPorts=6
  wires:
  Frequency Error/1 -> Voltage and Frequency Matching/4
  In1/1 -> Bus Creator3/1
  "Grid Active & Reactive Power "/2(Q) -> Bus Creator4/2  "Reactive Power (pu)"
  Grid Voltage/1 -> Bus Creator2/1
  Phase Angle Error/1 -> Voltage and Frequency Matching/5
  Island Angle/1 -> Bus Creator1/2
  Island Frequency/1 -> Bus Creator/2
  Voltage Error/1 -> Voltage and Frequency Matching/6
  Grid Angle/1 -> Bus Creator1/1
  Grid Frequency/1 -> Bus Creator/1
  Bus Creator/1 -> Voltage and Frequency Matching/1
  Bus Creator2/1 -> Voltage and Frequency Matching/3
  Bus Creator4/1 -> Resynch and PCC voltage,Current/4
  Grid Voltage abc/1 -> "Grid Active & Reactive Power "/1(Vabc), Resynch and PCC voltage,Current/3
  Island Voltage/1 -> Bus Creator2/2
  "Grid Active & Reactive Power "/1(P) -> Bus Creator4/1  "Active Power (pu)"
  Bus Creator3/1 -> Resynch and PCC voltage,Current/1
  Resynchronization/1 -> Bus Creator3/2
  Bus Creator1/1 -> Voltage and Frequency Matching/2
  Grid Current/1 -> "Grid Active & Reactive Power "/2(Iabc), Resynch and PCC voltage,Current/2

== system IndustrialMicrogrid/Operator Room/OperatorControlRoom/MG2 Controller : Commands and Measurements/Microgrid Controller 2 : Commands and Measurements/Monitoring of system performance/Load /Subsystem4 ==
  Voltage : Inport
  Change Detector : eeGeneralControl/Change Detector  VariantControl=Variant1  LabelModeActiveChoice=Discrete  ChangeType=Rising edge  x0=0  Ts=Ts
  Change Detector1 : eeGeneralControl/Change Detector  VariantControl=Variant1  LabelModeActiveChoice=Discrete  ChangeType=Rising edge  x0=0  Ts=Ts
  Compare To Constant2 : simulink/Logic and Bit Operations/Compare To Constant  relop=<=  const=microgrid.LoadVolatgeRMSLow  OutDataTypeStr=boolean
  Compare To Constant3 : simulink/Logic and Bit Operations/Compare To Constant  relop=>  const=microgrid.LoadVolatgeRMSHigh  OutDataTypeStr=boolean
  VoltageLow : Outport
  VoltageHigh : Outport  Port=2
  wires:
  Change Detector/1 -> VoltageLow/1
  Compare To Constant2/1 -> Change Detector/1
  Voltage/1 -> Compare To Constant3/1, Compare To Constant2/1
  Change Detector1/1 -> VoltageHigh/1
  Compare To Constant3/1 -> Change Detector1/1

== system IndustrialMicrogrid/Operator Room/OperatorControlRoom/MG2 Controller : Commands and Measurements/Microgrid Controller 2 : Commands and Measurements/Monitoring of system performance/Load /start at 0.2 s2 ==
  In1 : Inport
  Constant : Constant  Value=0.707
  Step : Step  Time=0.3  SampleTime=Ts
  Switch : Switch  Criteria=u2 > Threshold  Threshold=0.5  SaturateOnIntegerOverflow=off  InputSameDT=off
  u : Outport
  wires:
  In1/1 -> Switch/1
  Switch/1 -> u/1
  Constant/1 -> Switch/3
  Step/1 -> Switch/2

== system IndustrialMicrogrid/Operator Room/OperatorControlRoom/MG2 Controller : Commands and Measurements/Microgrid Controller 2 : Commands and Measurements/Monitoring of system performance/Load /start at 0.2 s4 ==
  In1 : Inport
  Constant : Constant  Value=0.491
  Step : Step  Time=0.3  SampleTime=Ts
  Switch : Switch  Criteria=u2 > Threshold  Threshold=0.5  SaturateOnIntegerOverflow=off  InputSameDT=off
  u : Outport
  wires:
  In1/1 -> Switch/1
  Switch/1 -> u/1
  Constant/1 -> Switch/3
  Step/1 -> Switch/2

== system IndustrialMicrogrid/Operator Room/OperatorControlRoom/MG2 Controller : Commands and Measurements/Microgrid Controller 2 : Commands and Measurements/Monitoring of system performance/Load /start at 0.2 s5 ==
  In1 : Inport
  Constant : Constant  Value=75
  Step : Step  Time=0.3  SampleTime=Ts
  Switch : Switch  Criteria=u2 > Threshold  Threshold=0.5  SaturateOnIntegerOverflow=off  InputSameDT=off
  u : Outport
  wires:
  Step/1 -> Switch/2
  Constant/1 -> Switch/3
  Switch/1 -> u/1
  In1/1 -> Switch/1

== system IndustrialMicrogrid/Operator Room/OperatorControlRoom/MG2 Controller : Commands and Measurements/Microgrid Controller 2 : Commands and Measurements/Monitoring of system performance/Microgrid/Subsystem ==
  Frequency : Inport
  Change Detector : eeGeneralControl/Change Detector  VariantControl=Variant1  LabelModeActiveChoice=Discrete  ChangeType=Rising edge  x0=0  Ts=Ts
  Change Detector1 : eeGeneralControl/Change Detector  VariantControl=Variant1  LabelModeActiveChoice=Discrete  ChangeType=Rising edge  x0=0  Ts=Ts
  Compare To Constant2 : simulink/Logic and Bit Operations/Compare To Constant  relop=<  const=(1-microgrid.FrequencyLimit1)*60  OutDataTypeStr=boolean
  Compare To Constant3 : simulink/Logic and Bit Operations/Compare To Constant  relop=>  const=(1+microgrid.FrequencyLimit1)*60  OutDataTypeStr=boolean
  FrequencyLow : Outport
  FrequencyHigh : Outport  Port=2
  wires:
  Change Detector/1 -> FrequencyLow/1
  Compare To Constant2/1 -> Change Detector/1
  Frequency/1 -> Compare To Constant3/1, Compare To Constant2/1
  Change Detector1/1 -> FrequencyHigh/1
  Compare To Constant3/1 -> Change Detector1/1

== system IndustrialMicrogrid/Operator Room/OperatorControlRoom/MG2 Controller : Commands and Measurements/Microgrid Controller 2 : Commands and Measurements/Monitoring of system performance/Microgrid/Subsystem3 ==
  Voltage : Inport
  Change Detector : eeGeneralControl/Change Detector  VariantControl=Variant1  LabelModeActiveChoice=Discrete  ChangeType=Rising edge  x0=0  Ts=Ts
  Change Detector1 : eeGeneralControl/Change Detector  VariantControl=Variant1  LabelModeActiveChoice=Discrete  ChangeType=Rising edge  x0=0  Ts=Ts
  Compare To Constant2 : simulink/Logic and Bit Operations/Compare To Constant  relop=<=  const=1-microgrid.VoltageLimit1  OutDataTypeStr=boolean
  Compare To Constant3 : simulink/Logic and Bit Operations/Compare To Constant  relop=>  const=1+microgrid.VoltageLimit1  OutDataTypeStr=boolean
  VoltageLow : Outport
  VoltageHigh : Outport  Port=2
  wires:
  Compare To Constant3/1 -> Change Detector/1
  Change Detector/1 -> VoltageHigh/1
  Voltage/1 -> Compare To Constant2/1, Compare To Constant3/1
  Compare To Constant2/1 -> Change Detector1/1
  Change Detector1/1 -> VoltageLow/1

== system IndustrialMicrogrid/Operator Room/OperatorControlRoom/MG2 Controller : Commands and Measurements/Microgrid Controller 2 : Commands and Measurements/Monitoring of system performance/Microgrid/start at 2 s ==
  In1 : Inport
  Constant : Constant  Value=60
  Step : Step  Time=2  SampleTime=Ts
  Switch : Switch  Criteria=u2 > Threshold  Threshold=0.5  SaturateOnIntegerOverflow=off  InputSameDT=off
  u : Outport
  wires:
  Step/1 -> Switch/2
  Constant/1 -> Switch/3
  Switch/1 -> u/1
  In1/1 -> Switch/1

== system IndustrialMicrogrid/Operator Room/OperatorControlRoom/MG2 Controller : Commands and Measurements/Microgrid Controller 2 : Commands and Measurements/Monitoring of system performance/Microgrid/start at 2 s1 ==
  In1 : Inport
  Constant : Constant
  Step : Step  Time=2  SampleTime=Ts
  Switch : Switch  Criteria=u2 > Threshold  Threshold=0.5  SaturateOnIntegerOverflow=off  InputSameDT=off
  u : Outport
  wires:
  Step/1 -> Switch/2
  Constant/1 -> Switch/3
  Switch/1 -> u/1
  In1/1 -> Switch/1

== system IndustrialMicrogrid/Operator Room/OperatorControlRoom/MG2 Controller : Commands and Measurements/Microgrid Controller 2 : Commands and Measurements/Monitoring of system performance/Subsystem/start at 2.5 s ==
  ReactivePower : Inport
  Constant : Constant  Value=0
  Step : Step  Time=2.5  SampleTime=Ts
  Switch : Switch  Criteria=u2 > Threshold  Threshold=0.5  SaturateOnIntegerOverflow=off  InputSameDT=off
  u : Outport
  wires:
  ReactivePower/1 -> Switch/1
  Switch/1 -> u/1
  Constant/1 -> Switch/3
  Step/1 -> Switch/2

== system IndustrialMicrogrid/Operator Room/OperatorControlRoom/MG2 Controller : Commands and Measurements/Microgrid Controller 2 : Commands and Measurements/Monitoring of system performance/Subsystem/start at 2.5 s1 ==
  ActivePower : Inport
  Constant : Constant  Value=0
  Step : Step  Time=2.5  SampleTime=Ts
  Switch : Switch  Criteria=u2 > Threshold  Threshold=0.5  SaturateOnIntegerOverflow=off  InputSameDT=off
  u : Outport
  wires:
  Step/1 -> Switch/2
  Constant/1 -> Switch/3
  Switch/1 -> u/1
  ActivePower/1 -> Switch/1

== system IndustrialMicrogrid/MG1 Primary Substation/BESS and Controller/BESS/Grid-Forming Converter Control/Current Limiting/CurrentLimitingMethod/currentLimitAndVirtual/Current Saturation ==
  note: Vs-delV
  Id : Inport
  Iq : Inport  Port=2
  Imaxsat : Inport  Port=3
  Enable : EnablePort
  Compare : Subsystem
  Constant1 : Constant  Value=0
  Constant2 : Constant  Value=0
  If : If
  If Action Subsystem : Subsystem  TreatAsAtomicUnit=on
  If Action Subsystem1 : Subsystem  TreatAsAtomicUnit=on
  Math Function : Math  Operator=hypot
  Merge : Merge
  Merge1 : Merge
  Subtract : Sum  Inputs=+-
  delVd : Outport
  delVq : Outport  Port=2
  idmax : Outport  Port=3
  iqmax : Outport  Port=4
  wires:
  Iq/1 -> [Isq], Math Function/2
  If/1 -> If Action Subsystem/Action
  If Action Subsystem1/1(Idmax) -> Merge/2
  Constant2/1 -> delVq/1
  Math Function/1 -> [Is], Subtract/2
  If/2 -> If Action Subsystem1/Action
  If Action Subsystem/2(Iqmax) -> Merge1/1
  Subtract/1 -> Compare/1(u)
  Compare/1(Out1) -> If/1
  If Action Subsystem/1(Idmax) -> Merge/1
  [Is] -> If Action Subsystem/1(Is)
  Id/1 -> [Isd], Math Function/1
  If Action Subsystem1/2(Iqmax) -> Merge1/2
  Merge/1 -> idmax/1
  [Isd] -> If Action Subsystem/2(Isd)
  Constant1/1 -> delVd/1
  [Isq] -> If Action Subsystem/3(Isq)
  Merge1/1 -> iqmax/1
  Imaxsat/1 -> [Imax], Subtract/1
  [Imax] -> If Action Subsystem/4(maxI)

== system IndustrialMicrogrid/MG1 Primary Substation/BESS and Controller/BESS/Grid-Forming Converter Control/Current Limiting/CurrentLimitingMethod/currentLimitAndVirtual/No Fault Ride Through ==
  Id : Inport
  Iq : Inport  Port=2
  Enable : EnablePort
  Constant{1..4} (4 alike) : Constant  Value=0
  Terminator : Terminator
  Terminator1 : Terminator
  delVd : Outport
  delVq : Outport  Port=2
  idmax : Outport  Port=3
  iqmax : Outport  Port=4
  wires:
  Constant3/1 -> iqmax/1
  Constant2/1 -> idmax/1
  Constant1/1 -> delVd/1
  Constant4/1 -> delVq/1
  Id/1 -> Terminator/1
  Iq/1 -> Terminator1/1

== system IndustrialMicrogrid/MG1 Primary Substation/BESS and Controller/BESS/Grid-Forming Converter Control/Current Limiting/CurrentLimitingMethod/currentLimitAndVirtual/VI ==
  note: Resistance coefficient
  note: X/R ratio
  Id : Inport
  Iq : Inport  Port=2
  Imax : Inport  Port=3
  Enable : EnablePort
  Constant1 : Constant  Value=0
  Constant2 : Constant  Value=0
  Constant3 : Constant  Value=0
  Gain : Gain  Gain=ctLimitVirtualImp
  Gain1 : Gain  Gain=ctLimitXbyR
  Low-Pass Filter : eeGeneralControl/Low-Pass Filter (Discrete or Continuous)  K=1  T=currentVITimeConst  B=inf  A=-inf  init_option=Inherited from block input  x0=0  Ts=-1
  Math Function : Math  Operator=hypot
  Product{,1..3} (4 alike) : Product
  Relay1 : Relay  OnSwitchValue=0.01  OffSwitchValue=-0.1
  Saturation : Saturate  UpperLimit=1  LowerLimit=-1
  Saturation1 : Saturate  UpperLimit=1  LowerLimit=-1
  Sum : Sum  Inputs=|+-
  Sum1 : Sum  Inputs=|+-
  Sum2 : Sum  Inputs=++|
  Switch : Switch  Criteria=u2 > Threshold  SaturateOnIntegerOverflow=off  InputSameDT=off
  delVd : Outport
  delVq : Outport  Port=2
  idmax : Outport  Port=3
  iqmax : Outport  Port=4
  wires:
  Gain1/1 -> Product1/2, Product2/1
  Product3/1 -> Sum2/2
  Id/1 -> Math Function/1, [Igd]
  Sum2/1 -> Saturation1/1
  Sum/1 -> Gain/1, Relay1/1
  Sum1/1 -> Saturation/1
  Product/1 -> Sum1/1
  [Igq] -> Product3/1, Product2/2
  Iq/1 -> [Igq], Math Function/2
  Math Function/1 -> Low-Pass Filter/1  "Is"
  Switch/1 -> Product3/2, Product/1, Gain1/1
  [Igd] -> Product1/1, Product/2
  Saturation1/1 -> delVq/1
  Product1/1 -> Sum2/1
  Product2/1 -> Sum1/2
  Gain/1 -> Switch/1
  Constant1/1 -> Switch/3
  Saturation/1 -> delVd/1
  Constant3/1 -> iqmax/1
  Constant2/1 -> idmax/1
  Relay1/1 -> Switch/2
  Low-Pass Filter/1 -> Sum/1
  Imax/1 -> Sum/2  "IsMaximum"

== system IndustrialMicrogrid/MG1 Primary Substation/BESS and Controller/BESS/Grid-Forming Converter Control/Current Limiting/CurrentLimitingMethod/currentSaturation/Compare ==
  u : Inport
  AND : Logic  IconShape=distinctive  AllPortsSameDT=off  OutDataTypeStr=boolean
  Compare To Constant : simulink/Logic and Bit Operations/Compare To Constant  relop=>  const=ctLimitDelayTime  OutDataTypeStr=boolean
  Compare To Zero : simulink/Logic and Bit Operations/Compare To Zero  relop=<=  OutDataTypeStr=boolean
  Data Type Conversion : DataTypeConversion  SaturateOnIntegerOverflow=off  RndMeth=Floor
  Data Type Conversion1 : DataTypeConversion  SaturateOnIntegerOverflow=off  RndMeth=Floor
  Discrete-Time Integrator : DiscreteIntegrator  IntegratorMethod=Integration: Backward Euler  ExternalReset=level  SampleTime=currentControlTs  LimitOutput=on  UpperSaturationLimit=ctLimitDelayTime*2  LowerSaturationLimit=0  ICPrevOutput=DiscIntNeverNeededParam  ICPrevScaledInput=DiscIntNeverNeededParam
  Out1 : Outport
  wires:
  AND/1 -> Data Type Conversion/1
  Compare To Zero/1 -> Data Type Conversion1/1
  Compare To Constant/1 -> AND/2
  u/1 -> Compare To Zero/1
  Discrete-Time Integrator/1 -> Compare To Constant/1
  Data Type Conversion/1 -> Out1/1
  Data Type Conversion1/1 -> Discrete-Time Integrator/2, Discrete-Time Integrator/1, AND/1
